simulink model "SerialReceivev1_1"  (R2015b)
settings: Solver=VariableStepAuto  StartTime=0.0  StopTime=inf  RelTol=1e-3
undefined symbols (not defined in the file or in its folder): LF, serial
libraries: instrumentlib x2, xpcseriallib x1
settings Model: Creator=TOOsab  LastModifiedBy=TOOsab

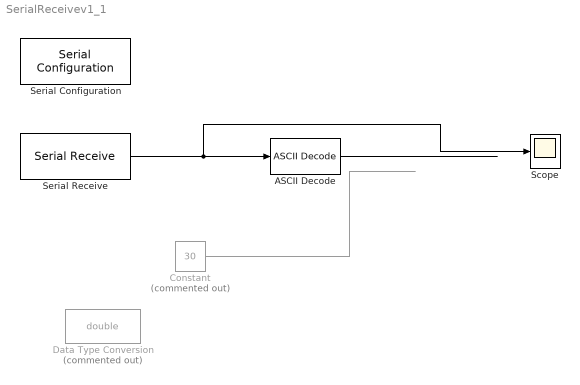
== system SerialReceivev1_1 ==
  "ASCII Decode " : xpcseriallib/ASCII Decode   format=%i\n  nvars=1  vartypes={}
  Constant : Constant  Commented=on  Value=30
  Data Type Conversion : DataTypeConversion  Commented=on  OutDataTypeStr=double
  Scope : Scope
  Serial Configuration : instrumentlib/Serial Configuration  Priority=-200000  ComPortMenu=COM4  ComPort=COM4  ObjConstructor=serial('COM4');  BaudRate=256000  DataBits=8  Parity=none  StopBits=1  FlowControl=none  Timeout=10  ByteOrder=LittleEndian
  Serial Receive : instrumentlib/Serial Receive  ComPortMenu=COM4  ComPort=COM4  ObjConstructor=serial('COM4');  Terminator=LF ('\n')  DataSize="[1  1]"  DataType=int8  EnableBlockingMode=on  ActionDataUnavailable=Output last received value  CustomValue=0  SampleTime=0.01
  wires:
  Constant/1 -> ?
  Serial Receive/1 -> Scope/1, "ASCII Decode "/1
  "ASCII Decode "/1 -> ?
